simulink model "s_2dsfl_pos_cntrl"  (Simulink 7.0)
settings: Solver=ode1  StartTime=0.0  StopTime=15  FixedStep=0.002  RelTol=1e-3
values from neighbouring files (symbols this model uses):
  A1 = A    [setup_2dsfl.m]
  A2 = A    [setup_2dsfl.m]
  B1 = B    [setup_2dsfl.m]
  B2 = B    [setup_2dsfl.m]
  C1 = eye( 4 )    [setup_2dsfl.m]
  C2 = eye( 4 )    [setup_2dsfl.m]
  D1 = zeros( 4, 1 )    [setup_2dsfl.m]
  D2 = zeros( 4, 1 )    [setup_2dsfl.m]
undefined symbols (not defined in the file or in its folder): K1, K2, qc_get_step_size
libraries: simulink_extras x6, simulink x2, quarc_library x2
settings Model: Creator=MLevis  LastModifiedBy=MLevis  ExtModeTrigDuration=5000
settings SolverCC: PositivePriorityOrder=on
settings RTWCC: SystemTargetFile=quarc_windows.tlc  TemplateMakefile=quarc_default_tmf  Description=QUARC Win32 Target  ProcessScript=quarc_windows_make_rtw_hook
settings STFCustomTargetCC: TargetPreCompLibLocation=C:\DOCUME~1\ALLUSE~1\APPLIC~1\QUARC\lib\2007b\windows\release  GenFloatMathFcnCalls=ANSI_C  SystemTargetFile=quarc_windows.tlc
settings GRTTargetCC: TargetPreCompLibLocation=C:\DOCUME~1\ALLUSE~1\APPLIC~1\QUARC\lib\2007b\windows\release  CompOptLevelCompliant=off  MatFileLogging=off  ExtMode=on  ExtModeMexFile=quarc_comm

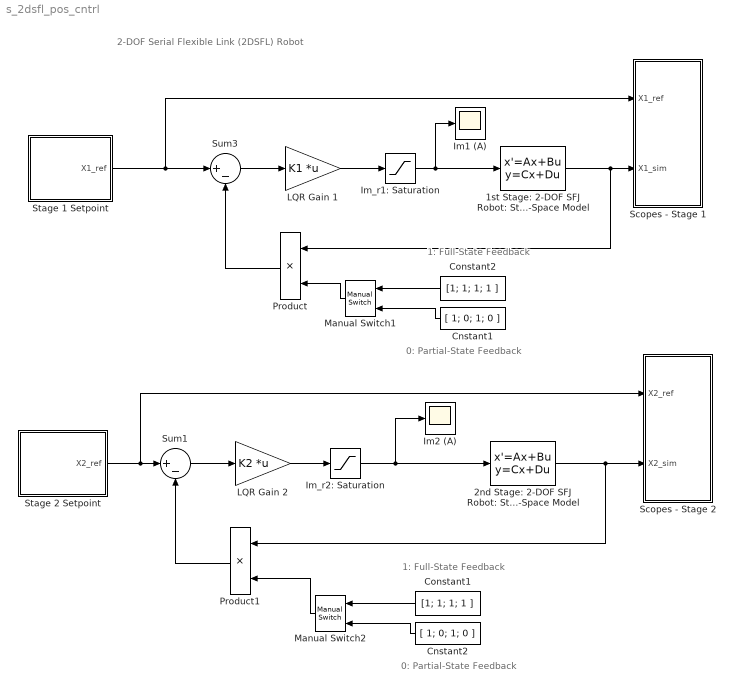
== system s_2dsfl_pos_cntrl ==
  note: 1: Full-State Feedback
  note: 0: Partial-State Feedback
  note: 1: Full-State Feedback
  note: 0: Partial-State Feedback
  note: 2-DOF Serial Flexible Link (2DSFL) Robot
  1st Stage: 2-DOF SFJ Robot: State-Space Model : StateSpace  A=A1  B=B1  C=C1  D=D1
  2nd Stage: 2-DOF SFJ Robot: State-Space Model : StateSpace  A=A2  B=B2  C=C2  D=D2
  Cnstant1 : Constant  Orientation=left  Value=[ 1; 0; 1; 0 ]  OutDataType=sfix(16)  OutScaling=2^0
  Cnstant2 : Constant  Orientation=left  Value=[ 1; 0; 1; 0 ]  OutDataType=sfix(16)  OutScaling=2^0
  Constant1 : Constant  Orientation=left  Value=[1; 1; 1; 1 ]  OutDataType=sfix(16)  OutScaling=2^0
  Constant2 : Constant  Orientation=left  Value=[1; 1; 1; 1 ]  OutDataType=sfix(16)  OutScaling=2^0
  Im1 (A) : Scope
      settings: TimeRange=15  YMin=-0.5  YMax=0.5
  Im2 (A) : Scope
      settings: TimeRange=15  YMin=-1.5  YMax=1.5  SaveName=ScopeData2
  Im_r1: Saturation : Saturate  UpperLimit=0.94  LowerLimit=-0.94
  Im_r2: Saturation : Saturate  UpperLimit=1.2  LowerLimit=-1.2
  LQR Gain 1 : Gain  Gain=K1  Multiplication=Matrix(K*u)  ParameterDataType=sfix(16)  ParameterScaling=2^0  OutDataType=sfix(16)  OutScaling=2^0
  LQR Gain 2 : Gain  Gain=K2  Multiplication=Matrix(K*u)  ParameterDataType=sfix(16)  ParameterScaling=2^0  OutDataType=sfix(16)  OutScaling=2^0
  Manual Switch1 : simulink/Signal Routing/Manual Switch  Orientation=left  SystemSampleTime=-1  sw=1  action=0  varsize=off
  Manual Switch2 : simulink/Signal Routing/Manual Switch  Orientation=left  SystemSampleTime=-1  sw=1  action=0  varsize=off
  Product : Product  Orientation=left  OutDataType=sfix(16)  OutScaling=2^0  SaturateOnIntegerOverflow=on  RndMeth=Zero  InputSameDT=on
  Product1 : Product  Orientation=left  OutDataType=sfix(16)  OutScaling=2^0  SaturateOnIntegerOverflow=on  RndMeth=Zero  InputSameDT=on
  Scopes - Stage 1 : Subsystem
  Scopes - Stage 2 : Subsystem
  Stage 1 Setpoint : Subsystem
  Stage 2 Setpoint : Subsystem
  Sum1 : Sum  Inputs=|+-  OutDataType=sfix(16)  OutScaling=2^0  SaturateOnIntegerOverflow=on  InputSameDT=on
  Sum3 : Sum  Inputs=|+-  OutDataType=sfix(16)  OutScaling=2^0  SaturateOnIntegerOverflow=on  InputSameDT=on
  wires:
  Constant2/1 -> Manual Switch1/1
  Cnstant1/1 -> Manual Switch1/2
  Manual Switch1/1 -> Product/2
  1st Stage: 2-DOF SFJ Robot: State-Space Model/1 -> Product/1, Scopes - Stage 1/2(X1_sim)
  Product/1 -> Sum3/2
  Stage 1 Setpoint/1(X1_ref) -> Sum3/1, Scopes - Stage 1/1(X1_ref)
  Sum3/1 -> LQR Gain 1/1
  LQR Gain 1/1 -> Im_r1: Saturation/1
  Im_r1: Saturation/1 -> 1st Stage: 2-DOF SFJ Robot: State-Space Model/1, Im1 (A)/1
  Product1/1 -> Sum1/2
  Sum1/1 -> LQR Gain 2/1
  Stage 2 Setpoint/1(X2_ref) -> Sum1/1, Scopes - Stage 2/1(X2_ref)
  LQR Gain 2/1 -> Im_r2: Saturation/1
  Im_r2: Saturation/1 -> 2nd Stage: 2-DOF SFJ Robot: State-Space Model/1, Im2 (A)/1
  2nd Stage: 2-DOF SFJ Robot: State-Space Model/1 -> Scopes - Stage 2/2(X2_sim), Product1/1
  Constant1/1 -> Manual Switch2/1
  Cnstant2/1 -> Manual Switch2/2
  Manual Switch2/1 -> Product1/2

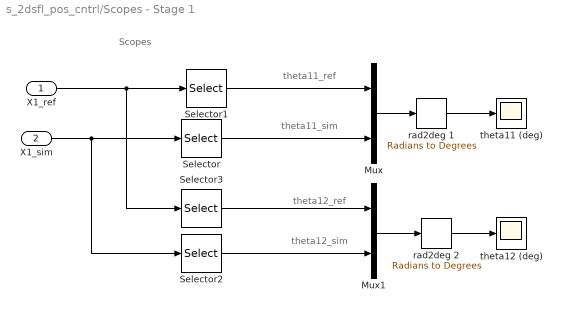
== system s_2dsfl_pos_cntrl/Scopes - Stage 1 ==
  note: theta11_sim
  note: theta11_ref
  note: theta12_sim
  note: Scopes
  note: theta12_ref
  X1_ref : Inport  OutDataType=sfix(16)  OutScaling=2^0
  X1_sim : Inport  Port=2  OutDataType=sfix(16)  OutScaling=2^0
  Mux : Mux  Inputs=2
  Mux1 : Mux  Inputs=2
  Selector : Selector  InputPortWidth=4  IndexOptions=Index vector (dialog)  Indices=[1]  OutputSizes=1
  Selector1 : Selector  InputPortWidth=4  IndexOptions=Index vector (dialog)  Indices=[1]  OutputSizes=1
  Selector2 : Selector  InputPortWidth=4  IndexOptions=Index vector (dialog)  Indices=[2]  OutputSizes=1
  Selector3 : Selector  InputPortWidth=4  IndexOptions=Index vector (dialog)  Indices=[2]  OutputSizes=1
  rad2deg 1 : simulink_extras/Transformations/Radians to Degrees  SystemSampleTime=-1
  rad2deg 2 : simulink_extras/Transformations/Radians to Degrees  SystemSampleTime=-1
  theta11 (deg) : Scope
      settings: TickLabels=on  TimeRange=15  YMin=-30  YMax=30  DataFormat=Array
  theta12 (deg) : Scope
      settings: TimeRange=15  YMin=-2  YMax=2  SaveName=data_th12  DataFormat=Array
  wires:
  Selector2/1 -> Mux1/2
  Selector/1 -> Mux/2
  rad2deg 2/1 -> theta12 (deg)/1
  rad2deg 1/1 -> theta11 (deg)/1
  X1_sim/1 -> Selector2/1, Selector/1
  Mux/1 -> rad2deg 1/1
  X1_ref/1 -> Selector1/1, Selector3/1
  Mux1/1 -> rad2deg 2/1
  Selector1/1 -> Mux/1
  Selector3/1 -> Mux1/1

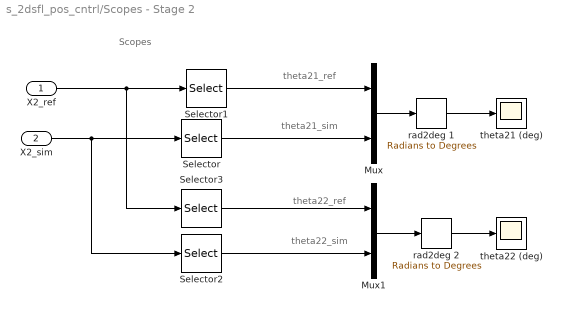
== system s_2dsfl_pos_cntrl/Scopes - Stage 2 ==
  note: theta22_ref
  note: Scopes
  note: theta22_sim
  note: theta21_ref
  note: theta21_sim
  X2_ref : Inport  OutDataType=sfix(16)  OutScaling=2^0
  X2_sim : Inport  Port=2  OutDataType=sfix(16)  OutScaling=2^0
  Mux : Mux  Inputs=2
  Mux1 : Mux  Inputs=2
  Selector : Selector  InputPortWidth=4  IndexOptions=Index vector (dialog)  Indices=[1]  OutputSizes=1
  Selector1 : Selector  InputPortWidth=4  IndexOptions=Index vector (dialog)  Indices=[1]  OutputSizes=1
  Selector2 : Selector  InputPortWidth=4  IndexOptions=Index vector (dialog)  Indices=[2]  OutputSizes=1
  Selector3 : Selector  InputPortWidth=4  IndexOptions=Index vector (dialog)  Indices=[2]  OutputSizes=1
  rad2deg 1 : simulink_extras/Transformations/Radians to Degrees  SystemSampleTime=-1
  rad2deg 2 : simulink_extras/Transformations/Radians to Degrees  SystemSampleTime=-1
  theta21 (deg) : Scope
      settings: TickLabels=on  TimeRange=15  YMin=-10  YMax=10  DataFormat=Array
  theta22 (deg) : Scope
      settings: TimeRange=15  YMin=-1  YMax=1  SaveName=data_th12  DataFormat=Array
  wires:
  Selector3/1 -> Mux1/1
  Selector1/1 -> Mux/1
  Mux1/1 -> rad2deg 2/1
  X2_ref/1 -> Selector3/1, Selector1/1
  Mux/1 -> rad2deg 1/1
  X2_sim/1 -> Selector/1, Selector2/1
  rad2deg 1/1 -> theta21 (deg)/1
  rad2deg 2/1 -> theta22 (deg)/1
  Selector/1 -> Mux/2
  Selector2/1 -> Mux1/2

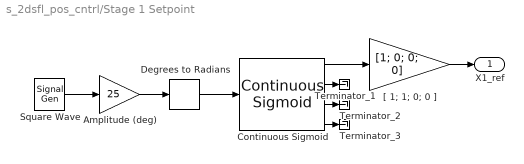
== system s_2dsfl_pos_cntrl/Stage 1 Setpoint ==
  Amplitude (deg) : Gain  Gain=25  ParameterDataType=sfix(16)  ParameterScaling=2^0  OutDataType=sfix(16)  OutScaling=2^0  SaturateOnIntegerOverflow=on
  Continuous Sigmoid : quarc_library/Sources/Sigmoids/Continuous Sigmoid  params_source=Internal (dialog parameters)  max_velocity=2.35  max_acceleration=4.45  initial_position=0  initial_velocity=0  hold_off=0.5  input_sample_time=-1  output_sample_time=qc_get_step_size
  Degrees to Radians : simulink_extras/Transformations/Degrees to Radians  SystemSampleTime=-1
  Square Wave : SignalGenerator  WaveForm=square  Frequency=0.1
  Terminator_1 : Terminator
  Terminator_2 : Terminator
  Terminator_3 : Terminator
  "[ 1; 1; 0; 0 ]" : Gain  Gain=[1; 0; 0; 0]  ParameterDataType=sfix(16)  ParameterScaling=2^0  OutDataType=sfix(16)  OutScaling=2^0  SaturateOnIntegerOverflow=on
  X1_ref : Outport
  wires:
  Square Wave/1 -> Amplitude (deg)/1
  Amplitude (deg)/1 -> Degrees to Radians/1
  "[ 1; 1; 0; 0 ]"/1 -> X1_ref/1
  Degrees to Radians/1 -> Continuous Sigmoid/1
  Continuous Sigmoid/2 -> Terminator_1/1
  Continuous Sigmoid/3 -> Terminator_2/1
  Continuous Sigmoid/4 -> Terminator_3/1
  Continuous Sigmoid/1 -> "[ 1; 1; 0; 0 ]"/1

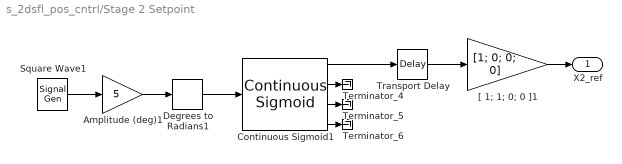
== system s_2dsfl_pos_cntrl/Stage 2 Setpoint ==
  Amplitude (deg)1 : Gain  Gain=5  ParameterDataType=sfix(16)  ParameterScaling=2^0  OutDataType=sfix(16)  OutScaling=2^0  SaturateOnIntegerOverflow=on
  Continuous Sigmoid1 : quarc_library/Sources/Sigmoids/Continuous Sigmoid  params_source=Internal (dialog parameters)  max_velocity=2  max_acceleration=5  initial_position=0  initial_velocity=0  hold_off=0.5  input_sample_time=-1  output_sample_time=qc_get_step_size
  Degrees to Radians1 : simulink_extras/Transformations/Degrees to Radians  SystemSampleTime=-1
  Square Wave1 : SignalGenerator  WaveForm=square  Frequency=0.1
  Terminator_4 : Terminator
  Terminator_5 : Terminator
  Terminator_6 : Terminator
  Transport Delay : TransportDelay  DelayTime=2.5  BufferSize=10/qc_get_step_size
  "[ 1; 1; 0; 0 ]1" : Gain  Gain=[1; 0; 0; 0]  ParameterDataType=sfix(16)  ParameterScaling=2^0  OutDataType=sfix(16)  OutScaling=2^0  SaturateOnIntegerOverflow=on
  X2_ref : Outport
  wires:
  Continuous Sigmoid1/1 -> Transport Delay/1
  Transport Delay/1 -> "[ 1; 1; 0; 0 ]1"/1
  Square Wave1/1 -> Amplitude (deg)1/1
  Amplitude (deg)1/1 -> Degrees to Radians1/1
  Continuous Sigmoid1/2 -> Terminator_4/1
  Continuous Sigmoid1/3 -> Terminator_5/1
  Continuous Sigmoid1/4 -> Terminator_6/1
  Degrees to Radians1/1 -> Continuous Sigmoid1/1
  "[ 1; 1; 0; 0 ]1"/1 -> X2_ref/1
